simulink model "practice2"  (R2014a)
settings: Solver=ode45  StartTime=0.0  StopTime=10.0  RelTol=1e-3
settings Model: Creator=Huanglei  LastModifiedBy=Huanglei

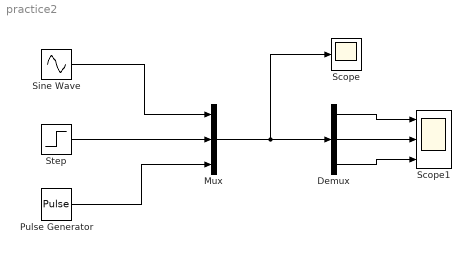
== system practice2 ==
  Demux : Demux  Outputs=3
  Mux : Mux  Inputs=3
  Pulse Generator : DiscretePulseGenerator  PulseType=Time based  Period=0.1  PulseWidth=50
  Scope : Scope
      settings: TimeRange=12
  Scope1 : Scope  NumInputPorts=3
      settings: YMin=-5~-5~-5  YMax=5~5~5
  Sine Wave : Sin  SampleTime=0
  Step : Step  SampleTime=0
  wires:
  Sine Wave/1 -> Mux/1
  Step/1 -> Mux/2
  Pulse Generator/1 -> Mux/3
  Mux/1 -> Scope/1, Demux/1
  Demux/1 -> Scope1/1
  Demux/3 -> Scope1/3
  Demux/2 -> Scope1/2
